simulink model "six_plus_six_AcmsteeringV09_main"  (R2014a)
settings: Solver=FixedStepDiscrete  StartTime=0.0  StopTime=10.0  FixedStep=0.0005  RelTol=1e-3
InitFcn:
  | Veh_Par_wxt
values from neighbouring files (symbols this model uses):
  acc_spdctl = [0 100]    [Veh_Par_wxt.m]
  ag_thr = ecucoder_cal(ag_thr)    [Veh_Par_wxt.m]
  B = 1.8    [Veh_Par_wxt.m]
  bra_em = 100    [Veh_Par_wxt.m]
  bra_pre_gz2 = 100/3    (= 33.3333333333)    [Veh_Par_wxt.m]
  bra_pre_gz34 = 10/3    (= 3.33333333333)    [Veh_Par_wxt.m]
  bra_pre_yd = 10/2    (= 5)    [Veh_Par_wxt.m]
  brakepre_dem_data = [0 1 2 3 4 5 6 7 8 9 10]    [Veh_Par_wxt.m]
  brakeTrq_dem_data = [0 125 251 376 502 627 753 878 1004 1129 1255]    [Veh_Par_wxt.m]
  bratrq_max = 4*1255    (= 5020)    [Veh_Par_wxt.m]
  eff_tran = 0.9    [Veh_Par_wxt.m]
  ESP_switch = ecucoder_cal(ESP_switch)    [Veh_Par_wxt.m]
  G = Mass*g    (= 15696)    [Veh_Par_wxt.m]
  kd1 = ecucoder_cal(kd1)    [Veh_Par_wxt.m]
  kd2 = 0    [Veh_Par_wxt.m]
  ki1 = ecucoder_cal(ki1)    [Veh_Par_wxt.m]
  ki2 = 1    [Veh_Par_wxt.m]
  kp1 = ecucoder_cal(kp1)    [Veh_Par_wxt.m]
  kp2 = 300    [Veh_Par_wxt.m]
  L = L1+L2    (= 2.9)    [Veh_Par_wxt.m]
  premax = 100    [Veh_Par_wxt.m]
  Radius = 0.4572/2    (= 0.2286)    [Veh_Par_wxt.m]
  RC_switch = ecucoder_cal(RC_switch)    [Veh_Par_wxt.m]
  s_opt_yi = 0.15    [Veh_Par_wxt.m]
  s_opt_zhuan = 0.8    [Veh_Par_wxt.m]
  s_opt_zhuan_add = 0.05    [Veh_Par_wxt.m]
  s_opt_zhuan_table = [0.8 0.8 0.3 0.3]    [Veh_Par_wxt.m]
  spd_map_mot = [0 499.85 999.79 1500 2000 2500 3000 3500 4000 4500 4999.8 5999.8]    [Veh_Par_wxt.m]
  spd_spdctl = [0 500]    [Veh_Par_wxt.m]
  speed_thr_park = 5/3.6/Radius*tras_ratio*30/pi    (= 464.143899364)    [Veh_Par_wxt.m]
  TCS_switch = ecucoder_cal(TCS_switch)    [Veh_Par_wxt.m]
  tras_ratio = 8    [Veh_Par_wxt.m]
  trq_map_mot = [70.5 70.012 71.154 65.797 53.917 45.159 38.073 32.685 27.48 17.133 14.949 10.07]    [Veh_Par_wxt.m]
  trqmax_yd = 70.5    [Veh_Par_wxt.m]
  trqmax_zx = 70.5    [Veh_Par_wxt.m]
  trqmaxneg = -70.5    [Veh_Par_wxt.m]
  v_gain = 0.9    [Veh_Par_wxt.m]
  v_table = [0 5 20 100]    [Veh_Par_wxt.m]
  v_thr_park = 5    [Veh_Par_wxt.m]
  zhidong_bianmazhi = [-140000 750000]    [Veh_Par_wxt.m]
  zhidong_down = -140000    [Veh_Par_wxt.m]
  zhidong_up = 750000    [Veh_Par_wxt.m]
  zhidong_youmen = [0 100]    [Veh_Par_wxt.m]
  zhuanxiang_bianmazhi = [-400000 0 400000]    [Veh_Par_wxt.m]
  zhuanxiang_down = -400000    [Veh_Par_wxt.m]
  zhuanxiang_up = 400000    [Veh_Par_wxt.m]
  zhuanxiang_youmen = [-100 0 100]    [Veh_Par_wxt.m]
undefined symbols (not defined in the file or in its folder): ecucoder_acal, guzhang_lf, guzhang_lm, guzhang_lr, guzhang_rf, guzhang_rm, guzhang_rr, myFIS
libraries: simulink x979, ec5744lib x59, fuzblock x2
(part 2 of 26)

== matlab function six_plus_six_AcmsteeringV09_main/MainControl/mode_control/backward/backward/Brake/Switch Case Action Subsystem/MATLAB Function5 ==
  data: bratrq_dem_lf input; bratrq_dem_lm input; bratrq_dem_lr input; bratrq_dem_rf input; bratrq_dem_rm input; bratrq_dem_rr input; pwr_chg_bat input; bratrq_mot_lf output; bratrq_mot_lm output; pwr_chg_bat1 input; pwr_chg_bat2 input; trqlimL_dig_lf input; bratrq_mot_lr output; bratrq_mot_rf output; bratrq_mot_rm output; bratrq_mot_rr output; trqlimL_dig_lm input; trqlimL_dig_lr input; trqlimL_dig_rf input; trqlimL_dig_rm input; trqlimL_dig_rr input; speed_act_lf input; speed_act_lm input; speed_act_lr input; speed_act_rf input; speed_act_rm input; speed_act_rr input; trqlim_map_lf input; brapre_out_l output; brapre_out_r output; trqlim_map_lm input; trqlim_map_lr input; trqlim_map_rf input; trqlim_map_rm input; trqlim_map_rr input; tras_ratio input; guzhang_lf input; guzhang_lm input; guzhang_lr input; guzhang_rf input; guzhang_rm input; guzhang_rr input
function [bratrq_mot_lf,bratrq_mot_lm,bratrq_mot_lr,bratrq_mot_rf,bratrq_mot_rm,bratrq_mot_rr,brapre_out_l,brapre_out_r] = fcn(bratrq_dem_lf,bratrq_dem_lm,bratrq_dem_lr,bratrq_dem_rf,bratrq_dem_rm,bratrq_dem_rr,pwr_chg_bat,pwr_chg_bat1,pwr_chg_bat2,trqlimL_dig_lf,trqlimL_dig_lm,trqlimL_dig_lr,trqlimL_dig_rf,trqlimL_dig_rm,trqlimL_dig_rr,speed_act_lf,speed_act_lm,speed_act_lr,speed_act_rf,speed_act_rm,speed_act_rr,trqlim_map_lf,trqlim_map_lm,trqlim_map_lr,trqlim_map_rf,trqlim_map_rm,trqlim_map_rr,tras_ratio,guzhang_lf,guzhang_lm,guzhang_lr,guzhang_rf,guzhang_rm,guzhang_rr)
%#codegen pid模块在外面做，里面进行十六种情况的判断，先看一下效果，不能再修改。前轴单独控制，后轴低选控制

bratrq_mot_lf1=single(bratrq_dem_lf/tras_ratio);
bratrq_mot_lf2=single(9549*(pwr_chg_bat/2)/speed_act_lf);
bratrq_mot_lf=single(min(trqlimL_dig_lf,min(bratrq_mot_lf1,bratrq_mot_lf2)));

bratrq_mot_lm1=single(bratrq_dem_lm/tras_ratio);
bratrq_mot_lm2=single(9549*(pwr_chg_bat1/2)/speed_act_lm);
bratrq_mot_lm=single(min(trqlimL_dig_lm,min(bratrq_mot_lm1,bratrq_mot_lm2)));

bratrq_mot_lr1=single(bratrq_dem_lr/tras_ratio);
bratrq_mot_lr2=single(9549*(pwr_chg_bat2/2)/speed_act_lr);
bratrq_mot_lr=single(min(trqlimL_dig_lr,min(bratrq_mot_lr1,bratrq_mot_lr2)));
 
bratrq_mot_rf1=single(bratrq_dem_rf/tras_ratio);
bratrq_mot_rf2=single(9549*(pwr_chg_bat/2)/speed_act_rf);
bratrq_mot_rf=single(min(trqlimL_dig_rf,min(bratrq_mot_rf1,bratrq_mot_rf2)));

bratrq_mot_rm1=single(bratrq_dem_rm/tras_ratio);
bratrq_mot_rm2=single(9549*(pwr_chg_bat1/2)/speed_act_rm);
bratrq_mot_rm=single(min(trqlimL_dig_rm,min(bratrq_mot_rm1,bratrq_mot_rm2)));

bratrq_mot_rr1=single(bratrq_dem_rr/tras_ratio);
bratrq_mot_rr2=single(9549*(pwr_chg_bat2/2)/speed_act_rr);
bratrq_mot_rr=single(min(trqlimL_dig_rr,min(bratrq_mot_rr1,bratrq_mot_rr2)));

brapre_out_l=single(((bratrq_dem_lf+bratrq_dem_lm+bratrq_dem_lr)-(bratrq_mot_lf+bratrq_mot_lm+bratrq_mot_lr)*tras_ratio)/3/150);
brapre_out_r=single(((bratrq_dem_rf+bratrq_dem_rm+bratrq_dem_rr)-(bratrq_mot_rf+bratrq_mot_rm+bratrq_mot_rr)*tras_ratio)/3/150);







bratrq_mot_lf=single(min(bratrq_mot_lf,trqlim_map_lf));%限一下最大值在外特性内，最小值大于0
bratrq_mot_lf=single(max(bratrq_mot_lf,0));
bratrq_mot_lr=single(min(bratrq_mot_lr,trqlim_map_lr));
bratrq_mot_lr=single(max(bratrq_mot_lr,0));
bratrq_mot_rf=single(min(bratrq_mot_rf,trqlim_map_rf));
bratrq_mot_rf=single(max(bratrq_mot_rf,0));
bratrq_mot_rr=single(min(bratrq_mot_rr,trqlim_map_rr));
bratrq_mot_rr=single(max(bratrq_mot_rr,0));

% brapre_out_l=brapre_out_l;
% brapre_out_r=brapre_out_r;
brapre_out_l=single(brapre_out_l*150/125);%第二辆车的制动压力与制动力的关系调整一下。
brapre_out_r=single(brapre_out_r*150/125);

if guzhang_lf==1
    bratrq_mot_lf=single(0);
end
if guzhang_lm==1
    bratrq_mot_lm=single(0);
end
if guzhang_lr==1
    bratrq_mot_lr=single(0);
end
if guzhang_rf==1
    bratrq_mot_rf=single(0);
end
if guzhang_rm==1
    bratrq_mot_rm=single(0);
end
if guzhang_rr==1
    bratrq_mot_rr=single(0);
end

end

== system six_plus_six_AcmsteeringV09_main/InputSignalProcess ==
  note: IMU坐标系转换到车辆坐标系
  note: 上坡辅助系统(Hill-start Assist Control，HAC)
  Signals : Inport
  function : TriggerPort  TriggerType=function-call
  Bus Creator : BusCreator  Inputs=8
  Bus Creator1 : BusCreator  Inputs=5
  Bus Creator2 : BusCreator  Inputs=17
  Bus Selector : BusSelector  OutputSignals=RemoteControl,MOTOR,CCM,motec,IMU
  Bus Selector1 : BusSelector  OutputSignals=RemoteControl1,RemoteControl2,RemoteControl3
  Bus Selector2 : BusSelector  OutputSignals=SE,LifeSpan,SH
  Bus Selector3 : BusSelector  OutputSignals=LeftJoystick_UpDown,LeftJoystick_LeftRight,RirhtJoystick_UpDown
  Bus Selector4 : BusSelector  OutputSignals=SA,SD
  Bus Selector6 : BusSelector  OutputSignals=IMU1.Xangularrate,IMU1.Yangularrate,IMU2.Zangularrate,IMU2.Xacceleration,IMU3.Yacceleration,IMU3.Zacceleration,IMU4.NorthSpd,IMU4.SkySpd,IMU5.EastSpd,IMU5.Altitude,IMU6.Longitude,IMU6.Latitude,IMU7.Rolling,IMU7.Heading,IMU8.Pitching
  Compare To Constant : simulink/Logic and Bit Operations/Compare To Constant  relop===  const=7  OutDataTypeStr=boolean
  Compare To Constant1 : simulink/Logic and Bit Operations/Compare To Constant  relop===  const=5  OutDataTypeStr=boolean
  Compare To Constant2 : simulink/Logic and Bit Operations/Compare To Constant  relop===  const=8  OutDataTypeStr=boolean
  Compare To Constant3 : simulink/Logic and Bit Operations/Compare To Constant  relop===  const=8  OutDataTypeStr=boolean
  Compare To Constant4 : simulink/Logic and Bit Operations/Compare To Constant  relop===  const=0  OutDataTypeStr=boolean
  Compare To Constant5 : simulink/Logic and Bit Operations/Compare To Constant  relop===  const=8  OutDataTypeStr=boolean
  Constant : Constant  Value=3  OutDataTypeStr=single  SampleTime=-1
  Constant1 : Constant  Value=0  OutDataTypeStr=single  SampleTime=-1
  Data Type Conversion{,1..16} (17 alike) : DataTypeConversion
  Dead Zone : DeadZone  LowerValue=-1  UpperValue=1  SaturateOnIntegerOverflow=on
  Dead Zone1 : DeadZone  LowerValue=-1  UpperValue=1  SaturateOnIntegerOverflow=on
  Dead Zone2 : DeadZone  LowerValue=0  UpperValue=3  SaturateOnIntegerOverflow=on
  Logical Operator : Logic  Operator=OR  Inputs=3  AllPortsSameDT=off  OutDataTypeStr=boolean
  MATLAB Function : MATLAB Function  TreatAsAtomicUnit=on
  MATLAB Function1 : MATLAB Function  TreatAsAtomicUnit=on
  Memory{,1..3} (4 alike) : Memory  InheritSampleTime=on
  Relational Operator : RelationalOperator  Operator===  OutDataTypeStr=boolean
  Terminator : Terminator
  Terminator1 : Terminator
  Signals_out : Outport
  wires:
  Signals/1 -> Bus Selector/1
  Bus Selector/1 -> Bus Selector1/1  "<RemoteControl>"
  Bus Selector1/1 -> Bus Selector2/1  "<RemoteControl1>"
  Bus Selector2/1 -> Compare To Constant1/1, Compare To Constant4/1, Compare To Constant/1  "<SE>"
  Bus Selector2/2 -> Relational Operator/1, Memory/1  "<LifeSpan>"
  Memory/1 -> Memory1/1
  Compare To Constant/1 -> Logical Operator/1
  Bus Selector1/2 -> Bus Selector3/1  "<RemoteControl2>"
  MATLAB Function/1(acc_dem) -> Dead Zone/1
  MATLAB Function/2(steer_dem) -> Dead Zone1/1
  MATLAB Function/3(brake_dem) -> Dead Zone2/1
  Logical Operator/1 -> Bus Creator/1  "brake_emerg"
  Compare To Constant1/1 -> Bus Creator/2  "park"
  Dead Zone/1 -> Bus Creator/3  "acc_dem"
  Dead Zone1/1 -> Bus Creator/4  "steer_dem"
  Dead Zone2/1 -> Bus Creator/5  "brake_dem"
  Bus Creator/1 -> Bus Creator1/1  "RemoteControl_dem"
  Bus Selector/2 -> Bus Creator1/2  "<MOTOR>"
  Bus Selector/3 -> Bus Creator1/3  "<CCM>"
  Bus Selector1/3 -> Bus Selector4/1  "<RemoteControl3>"
  Bus Selector4/1 -> Compare To Constant2/1  "<SA>"
  Compare To Constant2/1 -> Bus Creator/6  "center"
  Compare To Constant3/1 -> Bus Creator/7  "HAC"
  Bus Creator1/1 -> Signals_out/1
  Bus Selector/4 -> Bus Creator1/4  "<motec>"
  Memory1/1 -> Memory2/1
  Memory2/1 -> Memory3/1
  Memory3/1 -> Relational Operator/2
  Compare To Constant4/1 -> Logical Operator/2
  Compare To Constant5/1 -> Bus Creator/8  "SpdCtl_switch"
  Constant/1 -> Compare To Constant3/1
  Bus Selector2/3 -> Terminator/1  "<SH>"
  Bus Selector4/2 -> Compare To Constant5/1  "<SD>"
  Bus Selector3/3 -> MATLAB Function/3(RirhtJoystick_UpDown)  "<RirhtJoystick_UpDown>"
  Bus Selector3/1 -> MATLAB Function/1(LeftJoystick_UpDown)  "<LeftJoystick_UpDown>"
  Bus Selector3/2 -> MATLAB Function/2(LeftJoystick_LeftRight)  "<LeftJoystick_LeftRight>"
  Constant1/1 -> Logical Operator/3
  Relational Operator/1 -> Terminator1/1
  Bus Creator2/1 -> Bus Creator1/5  "IMU"
  Bus Selector/5 -> Bus Selector6/1  "<IMU>"
  Bus Selector6/1 -> MATLAB Function1/1(Xangularrate)  "<Xangularrate>"
  Bus Selector6/2 -> MATLAB Function1/2(Yangularrate)  "<Yangularrate>"
  Bus Selector6/5 -> MATLAB Function1/5(Yacceleration)  "<Yacceleration>"
  Bus Selector6/6 -> MATLAB Function1/6(Zacceleration)  "<Zacceleration>"
  Bus Selector6/10 -> MATLAB Function1/10(Altitude)  "<Altitude>"
  Bus Selector6/13 -> MATLAB Function1/13(Rolling)  "<Rolling>"
  Bus Selector6/15 -> MATLAB Function1/15(Pitching)  "<Pitching>"
  Bus Selector6/9 -> MATLAB Function1/9(EastSpd)  "<EastSpd>"
  Bus Selector6/12 -> MATLAB Function1/12(Latitude)  "<Latitude>"
  Bus Selector6/8 -> MATLAB Function1/8(SkySpd)  "<SkySpd>"
  Bus Selector6/14 -> MATLAB Function1/14(Heading)  "<Heading>"
  Bus Selector6/11 -> MATLAB Function1/11(Longitude)  "<Longitude>"
  Bus Selector6/4 -> MATLAB Function1/4(Xacceleration)  "<Xacceleration>"
  Bus Selector6/7 -> MATLAB Function1/7(NorthSpd)  "<NorthSpd>"
  Bus Selector6/3 -> MATLAB Function1/3(Zangularrate)  "<Zangularrate>"
  MATLAB Function1/6(Zacceleration1) -> Data Type Conversion5/1
  MATLAB Function1/2(Yangularrate1) -> Data Type Conversion1/1
  MATLAB Function1/7(NorthSpd1) -> Data Type Conversion6/1
  MATLAB Function1/4(Xacceleration1) -> Data Type Conversion3/1
  MATLAB Function1/5(Yacceleration1) -> Data Type Conversion4/1
  MATLAB Function1/10(Altitude1) -> Data Type Conversion9/1
  MATLAB Function1/8(SkySpd1) -> Data Type Conversion7/1
  MATLAB Function1/11(Longitude1) -> Data Type Conversion10/1
  MATLAB Function1/1(Xangularrate1) -> Data Type Conversion/1
  MATLAB Function1/3(Zangularrate1) -> Data Type Conversion2/1
  MATLAB Function1/13(Rolling1) -> Data Type Conversion12/1
  MATLAB Function1/12(Latitude1) -> Data Type Conversion11/1
  MATLAB Function1/9(EastSpd1) -> Data Type Conversion8/1
  MATLAB Function1/15(Pitching1) -> Data Type Conversion14/1
  MATLAB Function1/14(Heading1) -> Data Type Conversion13/1
  MATLAB Function1/17(Yspd) -> Data Type Conversion16/1  "Yspd"
  MATLAB Function1/16(Xspd) -> Data Type Conversion15/1  "Xspd"
  Data Type Conversion/1 -> Bus Creator2/1  "Xangularrate"
  Data Type Conversion1/1 -> Bus Creator2/2  "Yangularrate"
  Data Type Conversion2/1 -> Bus Creator2/3  "Zangularrate"
  Data Type Conversion3/1 -> Bus Creator2/4  "Xacceleration"
  Data Type Conversion4/1 -> Bus Creator2/5  "Yacceleration"
  Data Type Conversion5/1 -> Bus Creator2/6  "Zacceleration"
  Data Type Conversion6/1 -> Bus Creator2/7  "NorthSpd"
  Data Type Conversion7/1 -> Bus Creator2/8  "SkySpd"
  Data Type Conversion8/1 -> Bus Creator2/9  "EastSpd"
  Data Type Conversion9/1 -> Bus Creator2/10  "Altitude"
  Data Type Conversion10/1 -> Bus Creator2/11  "Longitude"
  Data Type Conversion11/1 -> Bus Creator2/12  "Latitude"
  Data Type Conversion12/1 -> Bus Creator2/13  "Rolling"
  Data Type Conversion13/1 -> Bus Creator2/14  "Heading"
  Data Type Conversion14/1 -> Bus Creator2/15  "Pitching"
  Data Type Conversion15/1 -> Bus Creator2/16  "Xspd"
  Data Type Conversion16/1 -> Bus Creator2/17  "Yspd"

== system six_plus_six_AcmsteeringV09_main/MainControl ==
  Signals : Inport
  function : TriggerPort  TriggerType=function-call
  mode_control : Subsystem
  mode_switch : Subsystem
  com_dem : Outport
  wires:
  Signals/1 -> mode_control/2(Signals), mode_switch/1(Signals)
  mode_switch/1(mode_dem_out) -> mode_control/1(mode_dem_out)
  mode_control/1(com_dem) -> com_dem/1

== system six_plus_six_AcmsteeringV09_main/Subsystem ==
  note: ID：电机1为201，电机2为202……
  note: ID：电机1为201，电机2为202……
  note: ID：电机1为201，电机2为202……
  note: ID：电机1为201，电机2为202……
  com_dem : Inport
  Trigger : TriggerPort  TriggerType=function-call  PortDimensions=1
  CANTransmit1 : ec5744lib/RapidECU_U3/04CANCommunication/CANTransmit  canmodule=0  canbuffer=10  canmessageid=hex2dec('C40F327')  canmessagetype=Extended(29-bit ID)  datalength=8  sampletime=-1
  CANTransmit11 : ec5744lib/RapidECU_U3/04CANCommunication/CANTransmit  canmodule=0  canbuffer=12  canmessageid=hex2dec('C40F027')  canmessagetype=Extended(29-bit ID)  datalength=8  sampletime=-1
  CANTransmit12 : ec5744lib/RapidECU_U3/04CANCommunication/CANTransmit  canmodule=0  canbuffer=11  canmessageid=hex2dec('C40F227')  canmessagetype=Extended(29-bit ID)  datalength=8  sampletime=-1
  CANTransmit2 : ec5744lib/RapidECU_U3/04CANCommunication/CANTransmit  canmodule=0  canbuffer=8  canmessageid=hex2dec('C40EF27')  canmessagetype=Extended(29-bit ID)  datalength=8  sampletime=-1
  CANTransmit4 : ec5744lib/RapidECU_U3/04CANCommunication/CANTransmit  canmodule=0  canbuffer=9  canmessageid=hex2dec('C40F127')  canmessagetype=Extended(29-bit ID)  datalength=8  sampletime=-1
  CANTransmit5 : ec5744lib/RapidECU_U3/04CANCommunication/CANTransmit  canmodule=0  canbuffer=13  canmessageid=hex2dec('C40F427')  canmessagetype=Extended(29-bit ID)  datalength=8  sampletime=-1
  CANTransmit6 : ec5744lib/RapidECU_U3/04CANCommunication/CANTransmit  canmodule=1  canbuffer=15  canmessageid=hex2dec('0202')  canmessagetype=Standard(11-bit ID)  datalength=6  sampletime=-1
  CANTransmit7 : ec5744lib/RapidECU_U3/04CANCommunication/CANTransmit  canmodule=1  canbuffer=56  canmessageid=hex2dec('0203')  canmessagetype=Standard(11-bit ID)  datalength=6  sampletime=-1
  CANTransmit8 : ec5744lib/RapidECU_U3/04CANCommunication/CANTransmit  canmodule=1  canbuffer=57  canmessageid=hex2dec('0204')  canmessagetype=Standard(11-bit ID)  datalength=6  sampletime=-1
  CANTransmit9 : ec5744lib/RapidECU_U3/04CANCommunication/CANTransmit  canmodule=1  canbuffer=58  canmessageid=hex2dec('0201')  canmessagetype=Standard(11-bit ID)  datalength=6  sampletime=-1
  Constant{2..3,6,8} (4 alike) : Constant  SampleTime=-1
  Constant{4..5,7,9} (4 alike) : Constant  Value=5  SampleTime=-1
  Data Type Conversion{,1..27} (28 alike) : DataTypeConversion
  Demux : Demux  Outputs=10
  Demux{1..6} (6 alike) : Demux  Outputs=6
  MATLAB Function : MATLAB Function  TreatAsAtomicUnit=on
  MATLAB Function1 : MATLAB Function  TreatAsAtomicUnit=on
  MATLAB Function2 : MATLAB Function  TreatAsAtomicUnit=on
  MATLAB Function3 : MATLAB Function  TreatAsAtomicUnit=on
  Memory{1..3,5} (4 alike) : Memory  InheritSampleTime=on  LinearizeAsDelay=on
  Mux{1..4} (4 alike) : Mux  Inputs=6
  Sum{1..8} (8 alike) : Sum  Inputs=|++
  Terminator{,1..8,10} (10 alike) : Terminator
  VCU1 : Subsystem
  VCU2 : Subsystem
  VCU3 : Subsystem
  VCU4 : Subsystem
  VCU5 : Subsystem
  VCU6 : Subsystem
  wires:
  VCU1/1(output) -> CANTransmit2/1
  CANTransmit2/1 -> Terminator/1
  VCU2/1(output) -> CANTransmit11/1
  CANTransmit11/1 -> Terminator1/1
  VCU3/1(output) -> CANTransmit4/1
  CANTransmit4/1 -> Terminator2/1
  VCU4/1(output) -> CANTransmit12/1
  CANTransmit12/1 -> Terminator3/1
  VCU5/1(output) -> CANTransmit1/1
  CANTransmit1/1 -> Terminator4/1
  VCU6/1(output) -> CANTransmit5/1
  CANTransmit5/1 -> Terminator5/1
  com_dem/1 -> Demux/1
  Demux/1 -> Demux1/1
  Demux1/2 -> VCU1/2(VCU1_CtrlModel_in)
  Demux1/1 -> VCU1/1(VCU1_EnableReq_in)
  Demux1/3 -> VCU1/3(VCU1_GearCmd_in)
  Demux1/4 -> VCU1/4(VCU1_SpeedMax_in)
  Demux1/5 -> VCU1/5(VCU1_TorqueRef_in)
  Demux1/6 -> VCU1/6(VCU1_LifeCnt_in)
  Demux/2 -> Demux2/1
  Demux2/1 -> VCU3/1(VCU1_EnableReq_in)
  Demux2/2 -> VCU3/2(VCU1_CtrlModel_in)
  Demux2/3 -> VCU3/3(VCU1_GearCmd_in)
  Demux2/5 -> VCU3/5(VCU1_TorqueRef_in)
  Demux2/6 -> VCU3/6(VCU1_LifeCnt_in)
  Demux2/4 -> VCU3/4(VCU1_SpeedMax_in)
  Demux3/5 -> VCU5/5(VCU1_TorqueRef_in)
  Demux3/6 -> VCU5/6(VCU1_LifeCnt_in)
  Demux3/4 -> VCU5/4(VCU1_SpeedMax_in)
  Demux3/2 -> VCU5/2(VCU1_CtrlModel_in)
  Demux3/1 -> VCU5/1(VCU1_EnableReq_in)
  Demux3/3 -> VCU5/3(VCU1_GearCmd_in)
  Demux/3 -> Demux3/1
  Demux4/1 -> VCU2/1(VCU1_EnableReq_in)
  Demux4/2 -> VCU2/2(VCU1_CtrlModel_in)
  Demux4/3 -> VCU2/3(VCU1_GearCmd_in)
  Demux4/4 -> VCU2/4(VCU1_SpeedMax_in)
  Demux4/5 -> VCU2/5(VCU1_TorqueRef_in)
  Demux4/6 -> VCU2/6(VCU1_LifeCnt_in)
  Demux/4 -> Demux4/1
  Demux5/3 -> VCU4/3(VCU1_GearCmd_in)
  Demux5/6 -> VCU4/6(VCU1_LifeCnt_in)
  Demux5/5 -> VCU4/5(VCU1_TorqueRef_in)
  Demux5/2 -> VCU4/2(VCU1_CtrlModel_in)
  Demux5/1 -> VCU4/1(VCU1_EnableReq_in)
  Demux5/4 -> VCU4/4(VCU1_SpeedMax_in)
  Demux6/4 -> VCU6/4(VCU1_SpeedMax_in)
  Demux6/1 -> VCU6/1(VCU1_EnableReq_in)
  Demux6/3 -> VCU6/3(VCU1_GearCmd_in)
  Demux6/6 -> VCU6/6(VCU1_LifeCnt_in)
  Demux6/2 -> VCU6/2(VCU1_CtrlModel_in)
  Demux6/5 -> VCU6/5(VCU1_TorqueRef_in)
  Demux/5 -> Demux5/1
  Demux/6 -> Demux6/1
  MATLAB Function/5(position_2) -> Data Type Conversion12/1
  Data Type Conversion2/1 -> Mux1/1
  Constant4/1 -> Sum1/1
  Memory5/1 -> Sum3/2
  Data Type Conversion6/1 -> Mux1/2
  CANTransmit6/1 -> Terminator10/1
  Constant2/1 -> Sum3/1
  MATLAB Function/6(position_1) -> Data Type Conversion9/1
  MATLAB Function/2(zero) -> Data Type Conversion6/1
  Mux1/1 -> CANTransmit6/1
  Sum1/1 -> MATLAB Function/1(data_1)
  MATLAB Function/1(data) -> Data Type Conversion2/1
  MATLAB Function/4(position_3) -> Data Type Conversion14/1
  MATLAB Function/3(position_4) -> Data Type Conversion10/1
  Sum3/1 -> Sum1/2, Memory5/1
  Data Type Conversion10/1 -> Mux1/3
  Data Type Conversion9/1 -> Mux1/6
  Data Type Conversion14/1 -> Mux1/4
  Data Type Conversion12/1 -> Mux1/5
  MATLAB Function1/5(position_2) -> Data Type Conversion3/1
  Data Type Conversion5/1 -> Mux2/1
  Constant5/1 -> Sum2/1
  Memory1/1 -> Sum4/2
  Data Type Conversion7/1 -> Mux2/2
  CANTransmit7/1 -> Terminator6/1
  Constant3/1 -> Sum4/1
  MATLAB Function1/6(position_1) -> Data Type Conversion8/1
  MATLAB Function1/2(zero) -> Data Type Conversion7/1
  Mux2/1 -> CANTransmit7/1
  Sum2/1 -> MATLAB Function1/1(data_1)
  MATLAB Function1/1(data) -> Data Type Conversion5/1
  MATLAB Function1/4(position_3) -> Data Type Conversion4/1
  MATLAB Function1/3(position_4) -> Data Type Conversion1/1
  Sum4/1 -> Memory1/1, Sum2/2
  Data Type Conversion1/1 -> Mux2/3
  Data Type Conversion8/1 -> Mux2/6
  Data Type Conversion4/1 -> Mux2/4
  Data Type Conversion3/1 -> Mux2/5
  MATLAB Function2/5(position_2) -> Data Type Conversion13/1
  Data Type Conversion16/1 -> Mux3/1
  Constant7/1 -> Sum5/1
  Memory2/1 -> Sum6/2
  Data Type Conversion17/1 -> Mux3/2
  CANTransmit8/1 -> Terminator7/1
  Constant6/1 -> Sum6/1
  MATLAB Function2/6(position_1) -> Data Type Conversion18/1
  MATLAB Function2/2(zero) -> Data Type Conversion17/1
  Mux3/1 -> CANTransmit8/1
  Sum5/1 -> MATLAB Function2/1(data_1)
  MATLAB Function2/1(data) -> Data Type Conversion16/1
  MATLAB Function2/4(position_3) -> Data Type Conversion15/1
  MATLAB Function2/3(position_4) -> Data Type Conversion11/1
  Sum6/1 -> Memory2/1, Sum5/2
  Data Type Conversion11/1 -> Mux3/3
  Data Type Conversion18/1 -> Mux3/6
  Data Type Conversion15/1 -> Mux3/4
  Data Type Conversion13/1 -> Mux3/5
  MATLAB Function3/5(position_2) -> Data Type Conversion20/1
  Data Type Conversion22/1 -> Mux4/1
  Constant9/1 -> Sum7/1
  Memory3/1 -> Sum8/2
  Data Type Conversion23/1 -> Mux4/2
  CANTransmit9/1 -> Terminator8/1
  Constant8/1 -> Sum8/1
  MATLAB Function3/6(position_1) -> Data Type Conversion24/1
  MATLAB Function3/2(zero) -> Data Type Conversion23/1
  Mux4/1 -> CANTransmit9/1
  Sum7/1 -> MATLAB Function3/1(data_1)
  MATLAB Function3/1(data) -> Data Type Conversion22/1
  MATLAB Function3/4(position_3) -> Data Type Conversion21/1
  MATLAB Function3/3(position_4) -> Data Type Conversion19/1
  Sum8/1 -> Memory3/1, Sum7/2
  Data Type Conversion19/1 -> Mux4/3
  Data Type Conversion24/1 -> Mux4/6
  Data Type Conversion21/1 -> Mux4/4
  Data Type Conversion20/1 -> Mux4/5
  Demux/9 -> Data Type Conversion26/1  "p3"
  Demux/7 -> Data Type Conversion/1
  Demux/10 -> Data Type Conversion27/1
  Data Type Conversion/1 -> MATLAB Function/2(data_2)
  Data Type Conversion25/1 -> MATLAB Function1/2(data_2)
  Data Type Conversion26/1 -> MATLAB Function2/2(data_2)
  Data Type Conversion27/1 -> MATLAB Function3/2(data_2)
  Demux/8 -> Data Type Conversion25/1

== system six_plus_six_AcmsteeringV09_main/Data_input/1 ==
  In1 : Inport
  In2 : Inport  Port=2
  function : TriggerPort  TriggerType=function-call
  Enabled Subsystem : Subsystem  TreatAsAtomicUnit=on
  motec_spd_2 : Outport
  motec_current_2 : Outport  Port=2
  enable_count : Outport  Port=3
  wires:
  In2/1 -> Enabled Subsystem/1(In2)
  In1/1 -> Enabled Subsystem/Enable
  Enabled Subsystem/1(motec_spd_2) -> motec_spd_2/1
  Enabled Subsystem/2(motec_current_2) -> motec_current_2/1
  Enabled Subsystem/3(enable_count2) -> enable_count/1

== system six_plus_six_AcmsteeringV09_main/Data_input/10 ==
  In1 : Inport
  In2 : Inport  Port=2
  function : TriggerPort  TriggerType=function-call
  Data Type Conversion : DataTypeConversion
  Data Type Conversion1 : DataTypeConversion
  Enabled Subsystem : Subsystem  TreatAsAtomicUnit=on
  Rolling_Out : Outport
  Heading_Out : Outport  Port=2
  wires:
  In1/1 -> Enabled Subsystem/Enable
  In2/1 -> Enabled Subsystem/1(In2)
  Enabled Subsystem/1(Rolling_Out) -> Data Type Conversion/1
  Enabled Subsystem/2(Heading_Out) -> Data Type Conversion1/1
  Data Type Conversion/1 -> Rolling_Out/1
  Data Type Conversion1/1 -> Heading_Out/1

== system six_plus_six_AcmsteeringV09_main/Data_input/11 ==
  In1 : Inport
  In2 : Inport  Port=2
  function : TriggerPort  TriggerType=function-call
  Data Type Conversion : DataTypeConversion
  Enabled Subsystem : Subsystem  TreatAsAtomicUnit=on
  Pitching_Out : Outport
  wires:
  In2/1 -> Enabled Subsystem/1(In2)
  In1/1 -> Enabled Subsystem/Enable
  Enabled Subsystem/1(Pitching_Out) -> Data Type Conversion/1
  Data Type Conversion/1 -> Pitching_Out/1

== system six_plus_six_AcmsteeringV09_main/Data_input/181 ==
  In1 : Inport
  In2 : Inport  Port=2
  function : TriggerPort  TriggerType=function-call
  Enabled Subsystem : Subsystem  TreatAsAtomicUnit=on
  motec_spd_1 : Outport
  motec_current_1 : Outport  Port=2
  enable_count1 : Outport  Port=3
  wires:
  In2/1 -> Enabled Subsystem/1(In2)
  In1/1 -> Enabled Subsystem/Enable
  Enabled Subsystem/1(motec_spd_1) -> motec_spd_1/1
  Enabled Subsystem/2(motec_current_1) -> motec_current_1/1
  Enabled Subsystem/3(enable_count1) -> enable_count1/1

== system six_plus_six_AcmsteeringV09_main/Data_input/2 ==
  In1 : Inport
  In2 : Inport  Port=2
  function : TriggerPort  TriggerType=function-call
  Enabled Subsystem : Subsystem  TreatAsAtomicUnit=on
  motec_spd_4 : Outport
  motec_current_4 : Outport  Port=2
  enable_count : Outport  Port=3
  wires:
  Enabled Subsystem/2(motec_current_4) -> motec_current_4/1
  Enabled Subsystem/1(motec_spd_4) -> motec_spd_4/1
  In1/1 -> Enabled Subsystem/Enable
  In2/1 -> Enabled Subsystem/1(In2)
  Enabled Subsystem/3(enable_count1) -> enable_count/1

== system six_plus_six_AcmsteeringV09_main/Data_input/3 ==
  In1 : Inport
  In2 : Inport  Port=2
  function : TriggerPort  TriggerType=function-call
  Enabled Subsystem : Subsystem  TreatAsAtomicUnit=on
  motec_spd_3 : Outport
  motec_current_3 : Outport  Port=2
  enable_count3 : Outport  Port=3
  wires:
  Enabled Subsystem/2(motec_current_3) -> motec_current_3/1
  Enabled Subsystem/1(motec_spd_3) -> motec_spd_3/1
  In1/1 -> Enabled Subsystem/Enable
  In2/1 -> Enabled Subsystem/1(In2)
  Enabled Subsystem/3(enable_count1) -> enable_count3/1

== system six_plus_six_AcmsteeringV09_main/Data_input/4 ==
  In1 : Inport
  In2 : Inport  Port=2
  function : TriggerPort  TriggerType=function-call
  Data Type Conversion : DataTypeConversion
  Data Type Conversion1 : DataTypeConversion
  Enabled Subsystem : Subsystem  TreatAsAtomicUnit=on
  Xangularrate_Out : Outport
  Yangularrate_Out : Outport  Port=2
  wires:
  In2/1 -> Enabled Subsystem/1(In2)
  In1/1 -> Enabled Subsystem/Enable
  Enabled Subsystem/1(Xangularrate_Out) -> Data Type Conversion/1
  Enabled Subsystem/2(Yangularrate_Out) -> Data Type Conversion1/1
  Data Type Conversion/1 -> Xangularrate_Out/1
  Data Type Conversion1/1 -> Yangularrate_Out/1

== system six_plus_six_AcmsteeringV09_main/Data_input/5 ==
  In1 : Inport
  In2 : Inport  Port=2
  function : TriggerPort  TriggerType=function-call
  Data Type Conversion : DataTypeConversion
  Data Type Conversion1 : DataTypeConversion
  Enabled Subsystem : Subsystem  TreatAsAtomicUnit=on
  Zangularrate_Out : Outport
  Xacceleration_Out : Outport  Port=2
  wires:
  Enabled Subsystem/2(Xacceleration_Out) -> Data Type Conversion1/1
  Enabled Subsystem/1(Zangularrate_Out) -> Data Type Conversion/1
  In1/1 -> Enabled Subsystem/Enable
  In2/1 -> Enabled Subsystem/1(In2)
  Data Type Conversion/1 -> Zangularrate_Out/1
  Data Type Conversion1/1 -> Xacceleration_Out/1

== system six_plus_six_AcmsteeringV09_main/Data_input/6 ==
  In1 : Inport
  In2 : Inport  Port=2
  function : TriggerPort  TriggerType=function-call
  Data Type Conversion : DataTypeConversion
  Data Type Conversion1 : DataTypeConversion
  Enabled Subsystem : Subsystem  TreatAsAtomicUnit=on
  Yacceleration_Out : Outport
  Zacceleration_Out : Outport  Port=2
  wires:
  In2/1 -> Enabled Subsystem/1(In2)
  In1/1 -> Enabled Subsystem/Enable
  Enabled Subsystem/1(Yacceleration_Out) -> Data Type Conversion/1
  Enabled Subsystem/2(Zacceleration_Out) -> Data Type Conversion1/1
  Data Type Conversion/1 -> Yacceleration_Out/1
  Data Type Conversion1/1 -> Zacceleration_Out/1

== system six_plus_six_AcmsteeringV09_main/Data_input/7 ==
  In1 : Inport
  In2 : Inport  Port=2
  function : TriggerPort  TriggerType=function-call
  Data Type Conversion : DataTypeConversion
  Data Type Conversion1 : DataTypeConversion
  Enabled Subsystem : Subsystem  TreatAsAtomicUnit=on
  NorthSpd_Out : Outport
  SkySpd_Out : Outport  Port=2
  wires:
  In1/1 -> Enabled Subsystem/Enable
  In2/1 -> Enabled Subsystem/1(In2)
  Enabled Subsystem/1(NorthSpd_Out) -> Data Type Conversion/1
  Enabled Subsystem/2(SkySpd_Out) -> Data Type Conversion1/1
  Data Type Conversion1/1 -> SkySpd_Out/1
  Data Type Conversion/1 -> NorthSpd_Out/1

== system six_plus_six_AcmsteeringV09_main/Data_input/8 ==
  In1 : Inport
  In2 : Inport  Port=2
  function : TriggerPort  TriggerType=function-call
  Data Type Conversion : DataTypeConversion
  Data Type Conversion1 : DataTypeConversion
  Enabled Subsystem : Subsystem  TreatAsAtomicUnit=on
  EastSpd_Out : Outport
  Altitude_Out : Outport  Port=2
  wires:
  Enabled Subsystem/2(Altitude_Out) -> Data Type Conversion1/1
  Enabled Subsystem/1(EastSpd_Out) -> Data Type Conversion/1
  In2/1 -> Enabled Subsystem/1(In2)
  In1/1 -> Enabled Subsystem/Enable
  Data Type Conversion1/1 -> Altitude_Out/1
  Data Type Conversion/1 -> EastSpd_Out/1

== system six_plus_six_AcmsteeringV09_main/Data_input/9 ==
  In1 : Inport
  In2 : Inport  Port=2
  function : TriggerPort  TriggerType=function-call
  Data Type Conversion : DataTypeConversion
  Data Type Conversion1 : DataTypeConversion
  Enabled Subsystem : Subsystem  TreatAsAtomicUnit=on
  Longitude_Out : Outport
  Latitude_Out : Outport  Port=2
  wires:
  In1/1 -> Enabled Subsystem/Enable
  In2/1 -> Enabled Subsystem/1(In2)
  Enabled Subsystem/1(Longitude_Out) -> Data Type Conversion/1
  Enabled Subsystem/2(Latitude_Out) -> Data Type Conversion1/1
  Data Type Conversion/1 -> Longitude_Out/1
  Data Type Conversion1/1 -> Latitude_Out/1

== system six_plus_six_AcmsteeringV09_main/Data_input/BMS1 ==
  In1 : Inport
  In2 : Inport  Port=2
  Trigger : TriggerPort  TriggerType=function-call  PortDimensions=1
  BMS1 : Subsystem
  BMS1_TotalVol : Outport
  BMS1_TotalCurrent : Outport  Port=2
  BMS1_Sys_Status2 : Outport  Port=3
  BMS1_Sys_Status1 : Outport  Port=4
  BMS1_SOC : Outport  Port=5
  wires:
  In2/1 -> BMS1/1(input)
  In1/1 -> BMS1/Enable
  BMS1/1(BMS1_TotalVol_Out) -> BMS1_TotalVol/1
  BMS1/4(BMS1_Sys_Status1_Out) -> BMS1_Sys_Status1/1
  BMS1/3(BMS1_Sys_Status2_Out) -> BMS1_Sys_Status2/1
  BMS1/5(BMS1_SOC_Out) -> BMS1_SOC/1
  BMS1/2(BMS1_TotalCurrent_Out) -> BMS1_TotalCurrent/1

== system six_plus_six_AcmsteeringV09_main/Data_input/BMS1-2 ==
  In1 : Inport
  In2 : Inport  Port=2
  Trigger : TriggerPort  TriggerType=function-call  PortDimensions=1
  BMS1 : Subsystem
  BMS1_TotalVol : Outport
  BMS1_TotalCurrent : Outport  Port=2
  BMS1_Sys_Status2 : Outport  Port=3
  BMS1_Sys_Status1 : Outport  Port=4
  BMS1_SOC : Outport  Port=5
  wires:
  In2/1 -> BMS1/1(input)
  In1/1 -> BMS1/Enable
  BMS1/1(BMS1_TotalVol_Out) -> BMS1_TotalVol/1
  BMS1/4(BMS1_Sys_Status1_Out) -> BMS1_Sys_Status1/1
  BMS1/3(BMS1_Sys_Status2_Out) -> BMS1_Sys_Status2/1
  BMS1/5(BMS1_SOC_Out) -> BMS1_SOC/1
  BMS1/2(BMS1_TotalCurrent_Out) -> BMS1_TotalCurrent/1

== system six_plus_six_AcmsteeringV09_main/Data_input/BMS1_1 ==
  In1 : Inport
  In2 : Inport  Port=2
  Trigger : TriggerPort  TriggerType=function-call  PortDimensions=1
  BMS1 : Subsystem
  BMS1_TotalVol : Outport
  BMS1_TotalCurrent : Outport  Port=2
  BMS1_Sys_Status2 : Outport  Port=3
  BMS1_Sys_Status1 : Outport  Port=4
  BMS1_SOC : Outport  Port=5
  wires:
  In2/1 -> BMS1/1(input)
  In1/1 -> BMS1/Enable
  BMS1/1(BMS1_TotalVol_Out) -> BMS1_TotalVol/1
  BMS1/4(BMS1_Sys_Status1_Out) -> BMS1_Sys_Status1/1
  BMS1/3(BMS1_Sys_Status2_Out) -> BMS1_Sys_Status2/1
  BMS1/5(BMS1_SOC_Out) -> BMS1_SOC/1
  BMS1/2(BMS1_TotalCurrent_Out) -> BMS1_TotalCurrent/1

== system six_plus_six_AcmsteeringV09_main/Data_input/BMS2 ==
  In1 : Inport
  In2 : Inport  Port=2
  Trigger : TriggerPort  TriggerType=function-call  PortDimensions=1
  BMS2 : Subsystem
  BMS2_LowSingleVol : Outport
  BMS2_HighSingleVol : Outport  Port=2
  wires:
  BMS2/2(BMS2_HighSingleVol_Out) -> BMS2_HighSingleVol/1
  BMS2/1(BMS2_LowSingleVol_Out) -> BMS2_LowSingleVol/1
  In1/1 -> BMS2/Enable
  In2/1 -> BMS2/1(input)

== system six_plus_six_AcmsteeringV09_main/Data_input/BMS2_1 ==
  In1 : Inport
  In2 : Inport  Port=2
  Trigger : TriggerPort  TriggerType=function-call  PortDimensions=1
  BMS2 : Subsystem
  BMS2_LowSingleVol : Outport
  BMS2_HighSingleVol : Outport  Port=2
  wires:
  BMS2/2(BMS2_HighSingleVol_Out) -> BMS2_HighSingleVol/1
  BMS2/1(BMS2_LowSingleVol_Out) -> BMS2_LowSingleVol/1
  In1/1 -> BMS2/Enable
  In2/1 -> BMS2/1(input)

== system six_plus_six_AcmsteeringV09_main/Data_input/BMS2_2 ==
  In1 : Inport
  In2 : Inport  Port=2
  Trigger : TriggerPort  TriggerType=function-call  PortDimensions=1
  BMS2 : Subsystem
  BMS2_LowSingleVol : Outport
  BMS2_HighSingleVol : Outport  Port=2
  wires:
  BMS2/2(BMS2_HighSingleVol_Out) -> BMS2_HighSingleVol/1
  BMS2/1(BMS2_LowSingleVol_Out) -> BMS2_LowSingleVol/1
  In1/1 -> BMS2/Enable
  In2/1 -> BMS2/1(input)

== system six_plus_six_AcmsteeringV09_main/Data_input/BMS3 ==
  In1 : Inport
  In2 : Inport  Port=2
  Trigger : TriggerPort  TriggerType=function-call  PortDimensions=1
  BMS3 : Subsystem
  BMS3_LowTemperature : Outport
  BMS3_HighTemperature : Outport  Port=2
  wires:
  In2/1 -> BMS3/1(input)
  BMS3/2(BMS3_HighTemperature_Out) -> BMS3_HighTemperature/1
  BMS3/1(BMS3_LowTemperature_Out) -> BMS3_LowTemperature/1
  In1/1 -> BMS3/Enable

== system six_plus_six_AcmsteeringV09_main/Data_input/BMS3_1 ==
  In1 : Inport
  In2 : Inport  Port=2
  Trigger : TriggerPort  TriggerType=function-call  PortDimensions=1
  BMS3 : Subsystem
  BMS3_LowTemperature : Outport
  BMS3_HighTemperature : Outport  Port=2
  wires:
  In2/1 -> BMS3/1(input)
  BMS3/2(BMS3_HighTemperature_Out) -> BMS3_HighTemperature/1
  BMS3/1(BMS3_LowTemperature_Out) -> BMS3_LowTemperature/1
  In1/1 -> BMS3/Enable

== system six_plus_six_AcmsteeringV09_main/Data_input/BMS3_2 ==
  In1 : Inport
  In2 : Inport  Port=2
  Trigger : TriggerPort  TriggerType=function-call  PortDimensions=1
  BMS3 : Subsystem
  BMS3_LowTemperature : Outport
  BMS3_HighTemperature : Outport  Port=2
  wires:
  In2/1 -> BMS3/1(input)
  BMS3/2(BMS3_HighTemperature_Out) -> BMS3_HighTemperature/1
  BMS3/1(BMS3_LowTemperature_Out) -> BMS3_LowTemperature/1
  In1/1 -> BMS3/Enable

== system six_plus_six_AcmsteeringV09_main/Data_input/BMS4 ==
  In1 : Inport
  In2 : Inport  Port=2
  Trigger : TriggerPort  TriggerType=function-call  PortDimensions=1
  BMS4 : Subsystem
  BMS4_Sys_Status : Outport
  BMS4_InputVolKEYON : Outport  Port=2
  BMS4_InputVolCHG : Outport  Port=3
  BMS4_InputVolACC : Outport  Port=4
  wires:
  In2/1 -> BMS4/1(input)
  BMS4/2(BMS4_InputVolKEYON_Out) -> BMS4_InputVolKEYON/1
  In1/1 -> BMS4/Enable
  BMS4/4(BMS4_InputVolACC_Out) -> BMS4_InputVolACC/1
  BMS4/1(BMS4_Sys_Status3_Out) -> BMS4_Sys_Status/1
  BMS4/3(BMS4_InputVolCHG_Out) -> BMS4_InputVolCHG/1

== system six_plus_six_AcmsteeringV09_main/Data_input/BMS4_1 ==
  In1 : Inport
  In2 : Inport  Port=2
  Trigger : TriggerPort  TriggerType=function-call  PortDimensions=1
  BMS4 : Subsystem
  BMS4_Sys_Status : Outport
  BMS4_InputVolKEYON : Outport  Port=2
  BMS4_InputVolCHG : Outport  Port=3
  BMS4_InputVolACC : Outport  Port=4
  wires:
  In2/1 -> BMS4/1(input)
  BMS4/2(BMS4_InputVolKEYON_Out) -> BMS4_InputVolKEYON/1
  In1/1 -> BMS4/Enable
  BMS4/4(BMS4_InputVolACC_Out) -> BMS4_InputVolACC/1
  BMS4/1(BMS4_Sys_Status3_Out) -> BMS4_Sys_Status/1
  BMS4/3(BMS4_InputVolCHG_Out) -> BMS4_InputVolCHG/1

== system six_plus_six_AcmsteeringV09_main/Data_input/BMS4_2 ==
  In1 : Inport
  In2 : Inport  Port=2
  Trigger : TriggerPort  TriggerType=function-call  PortDimensions=1
  BMS4 : Subsystem
  BMS4_Sys_Status : Outport
  BMS4_InputVolKEYON : Outport  Port=2
  BMS4_InputVolCHG : Outport  Port=3
  BMS4_InputVolACC : Outport  Port=4
  wires:
  In2/1 -> BMS4/1(input)
  BMS4/2(BMS4_InputVolKEYON_Out) -> BMS4_InputVolKEYON/1
  In1/1 -> BMS4/Enable
  BMS4/4(BMS4_InputVolACC_Out) -> BMS4_InputVolACC/1
  BMS4/1(BMS4_Sys_Status3_Out) -> BMS4_Sys_Status/1
  BMS4/3(BMS4_InputVolCHG_Out) -> BMS4_InputVolCHG/1

== system six_plus_six_AcmsteeringV09_main/Data_input/BMS5 ==
  In1 : Inport
  In2 : Inport  Port=2
  Trigger : TriggerPort  TriggerType=function-call  PortDimensions=1
  BMS5 : Subsystem
  BMS5_UpDownReuest : Outport
  BMS5_FeedbackPower : Outport  Port=2
  BMS5_FailureLevel : Outport  Port=3
  BMS5_ContDischargePower : Outport  Port=4
  BMS5_15s_InstanceDisPower : Outport  Port=5
  wires:
  BMS5/5(BMS5_15s_InstanceDisPower_Out) -> BMS5_15s_InstanceDisPower/1
  BMS5/1(BMS5_UpDownRequest_Out) -> BMS5_UpDownReuest/1
  In2/1 -> BMS5/1(input)
  BMS5/4(BMS5_ContDischargePower_Out) -> BMS5_ContDischargePower/1
  BMS5/2(BMS5_FeedbackPower_Out) -> BMS5_FeedbackPower/1
  BMS5/3(BMS5_FailureLevel_Out) -> BMS5_FailureLevel/1
  In1/1 -> BMS5/Enable

== system six_plus_six_AcmsteeringV09_main/Data_input/BMS5_1 ==
  In1 : Inport
  In2 : Inport  Port=2
  Trigger : TriggerPort  TriggerType=function-call  PortDimensions=1
  BMS5 : Subsystem
  BMS5_UpDownReuest : Outport
  BMS5_FeedbackPower : Outport  Port=2
  BMS5_FailureLevel : Outport  Port=3
  BMS5_ContDischargePower : Outport  Port=4
  BMS5_15s_InstanceDisPower : Outport  Port=5
  wires:
  BMS5/5(BMS5_15s_InstanceDisPower_Out) -> BMS5_15s_InstanceDisPower/1
  BMS5/1(BMS5_UpDownRequest_Out) -> BMS5_UpDownReuest/1
  In2/1 -> BMS5/1(input)
  BMS5/4(BMS5_ContDischargePower_Out) -> BMS5_ContDischargePower/1
  BMS5/2(BMS5_FeedbackPower_Out) -> BMS5_FeedbackPower/1
  BMS5/3(BMS5_FailureLevel_Out) -> BMS5_FailureLevel/1
  In1/1 -> BMS5/Enable

== system six_plus_six_AcmsteeringV09_main/Data_input/BMS5_2 ==
  In1 : Inport
  In2 : Inport  Port=2
  Trigger : TriggerPort  TriggerType=function-call  PortDimensions=1
  BMS5 : Subsystem
  BMS5_UpDownReuest : Outport
  BMS5_FeedbackPower : Outport  Port=2
  BMS5_FailureLevel : Outport  Port=3
  BMS5_ContDischargePower : Outport  Port=4
  BMS5_15s_InstanceDisPower : Outport  Port=5
  wires:
  BMS5/5(BMS5_15s_InstanceDisPower_Out) -> BMS5_15s_InstanceDisPower/1
  BMS5/1(BMS5_UpDownRequest_Out) -> BMS5_UpDownReuest/1
  In2/1 -> BMS5/1(input)
  BMS5/4(BMS5_ContDischargePower_Out) -> BMS5_ContDischargePower/1
  BMS5/2(BMS5_FeedbackPower_Out) -> BMS5_FeedbackPower/1
  BMS5/3(BMS5_FailureLevel_Out) -> BMS5_FailureLevel/1
  In1/1 -> BMS5/Enable

== system six_plus_six_AcmsteeringV09_main/Data_input/Enabled Subsystem ==
  In1 : Inport
  Enable : EnablePort
  Subsystem : Subsystem
  Out1 : Outport
  wires:
  In1/1 -> Out1/1

== system six_plus_six_AcmsteeringV09_main/Data_input/MCU0 ==
  In1 : Inport
  In2 : Inport  Port=2
  Trigger : TriggerPort  TriggerType=function-call  PortDimensions=1
  MCU0 : Subsystem
  MCU0_TorqueMax : Outport
  MCU0_EmergShutDown : Outport  Port=2
  MCU_ShutDownAllow : Outport  Port=3
  MCU_HighVol : Outport  Port=4
  MCU0_LiftCnt : Outport  Port=5
  MCU0_torqueFdk : Outport  Port=6
  MCU0_SpeedFdk : Outport  Port=7
  MCU0_GearStatus : Outport  Port=8
  MCU0_ControlMode : Outport  Port=9
  MCU0_WorkStatus : Outport  Port=10
  wires:
  In2/1 -> MCU0/1(input)
  In1/1 -> MCU0/Enable
  MCU0/1(MCU0_TorqueMax_Out) -> MCU0_TorqueMax/1
  MCU0/2(MCU0_EmergShutDown_Out) -> MCU0_EmergShutDown/1
  MCU0/5(MCU0_LiftCnt_Out) -> MCU0_LiftCnt/1
  MCU0/6(MCU0_TorqueFdk_Out) -> MCU0_torqueFdk/1
  MCU0/7(MCU0_SpeedFdk_Out) -> MCU0_SpeedFdk/1
  MCU0/3(MCU0_ShutDowAllow_Out) -> MCU_ShutDownAllow/1
  MCU0/4(MCU0_HighVol_Out) -> MCU_HighVol/1
  MCU0/10(MCU0_WorkStatus_Out) -> MCU0_WorkStatus/1
  MCU0/8(MCU0_GearStatus_Out) -> MCU0_GearStatus/1
  MCU0/9(MCU0_ControlMode_Out) -> MCU0_ControlMode/1

== system six_plus_six_AcmsteeringV09_main/Data_input/MCU0_1 ==
  In1 : Inport
  In2 : Inport  Port=2
  Trigger : TriggerPort  TriggerType=function-call  PortDimensions=1
  MCU0 : Subsystem
  MCU0_TorqueMax : Outport
  MCU0_EmergShutDown : Outport  Port=2
  MCU_ShutDownAllow : Outport  Port=3
  MCU_HighVol : Outport  Port=4
  MCU0_LiftCnt : Outport  Port=5
  MCU0_torqueFdk : Outport  Port=6
  MCU0_SpeedFdk : Outport  Port=7
  MCU0_GearStatus : Outport  Port=8
  MCU0_ControlMode : Outport  Port=9
  MCU0_WorkStatus : Outport  Port=10
  wires:
  In2/1 -> MCU0/1(input)
  In1/1 -> MCU0/Enable
  MCU0/1(MCU0_TorqueMax_Out) -> MCU0_TorqueMax/1
  MCU0/2(MCU0_EmergShutDown_Out) -> MCU0_EmergShutDown/1
  MCU0/5(MCU0_LiftCnt_Out) -> MCU0_LiftCnt/1
  MCU0/6(MCU0_TorqueFdk_Out) -> MCU0_torqueFdk/1
  MCU0/7(MCU0_SpeedFdk_Out) -> MCU0_SpeedFdk/1
  MCU0/3(MCU0_ShutDowAllow_Out) -> MCU_ShutDownAllow/1
  MCU0/4(MCU0_HighVol_Out) -> MCU_HighVol/1
  MCU0/10(MCU0_WorkStatus_Out) -> MCU0_WorkStatus/1
  MCU0/8(MCU0_GearStatus_Out) -> MCU0_GearStatus/1
  MCU0/9(MCU0_ControlMode_Out) -> MCU0_ControlMode/1

== system six_plus_six_AcmsteeringV09_main/Data_input/MCU0_2 ==
  In1 : Inport
  In2 : Inport  Port=2
  Trigger : TriggerPort  TriggerType=function-call  PortDimensions=1
  MCU0 : Subsystem
  MCU0_TorqueMax : Outport
  MCU0_EmergShutDown : Outport  Port=2
  MCU_ShutDownAllow : Outport  Port=3
  MCU_HighVol : Outport  Port=4
  MCU0_LiftCnt : Outport  Port=5
  MCU0_torqueFdk : Outport  Port=6
  MCU0_SpeedFdk : Outport  Port=7
  MCU0_GearStatus : Outport  Port=8
  MCU0_ControlMode : Outport  Port=9
  MCU0_WorkStatus : Outport  Port=10
  wires:
  In2/1 -> MCU0/1(input)
  In1/1 -> MCU0/Enable
  MCU0/1(MCU0_TorqueMax_Out) -> MCU0_TorqueMax/1
  MCU0/2(MCU0_EmergShutDown_Out) -> MCU0_EmergShutDown/1
  MCU0/5(MCU0_LiftCnt_Out) -> MCU0_LiftCnt/1
  MCU0/6(MCU0_TorqueFdk_Out) -> MCU0_torqueFdk/1
  MCU0/7(MCU0_SpeedFdk_Out) -> MCU0_SpeedFdk/1
  MCU0/3(MCU0_ShutDowAllow_Out) -> MCU_ShutDownAllow/1
  MCU0/4(MCU0_HighVol_Out) -> MCU_HighVol/1
  MCU0/10(MCU0_WorkStatus_Out) -> MCU0_WorkStatus/1
  MCU0/8(MCU0_GearStatus_Out) -> MCU0_GearStatus/1
  MCU0/9(MCU0_ControlMode_Out) -> MCU0_ControlMode/1

== system six_plus_six_AcmsteeringV09_main/Data_input/MCU0_3 ==
  In1 : Inport
  In2 : Inport  Port=2
  Trigger : TriggerPort  TriggerType=function-call  PortDimensions=1
  MCU0 : Subsystem
  MCU0_TorqueMax : Outport
  MCU0_EmergShutDown : Outport  Port=2
  MCU_ShutDownAllow : Outport  Port=3
  MCU_HighVol : Outport  Port=4
  MCU0_LiftCnt : Outport  Port=5
  MCU0_torqueFdk : Outport  Port=6
  MCU0_SpeedFdk : Outport  Port=7
  MCU0_GearStatus : Outport  Port=8
  MCU0_ControlMode : Outport  Port=9
  MCU0_WorkStatus : Outport  Port=10
  wires:
  In2/1 -> MCU0/1(input)
  In1/1 -> MCU0/Enable
  MCU0/1(MCU0_TorqueMax_Out) -> MCU0_TorqueMax/1
  MCU0/2(MCU0_EmergShutDown_Out) -> MCU0_EmergShutDown/1
  MCU0/5(MCU0_LiftCnt_Out) -> MCU0_LiftCnt/1
  MCU0/6(MCU0_TorqueFdk_Out) -> MCU0_torqueFdk/1
  MCU0/7(MCU0_SpeedFdk_Out) -> MCU0_SpeedFdk/1
  MCU0/3(MCU0_ShutDowAllow_Out) -> MCU_ShutDownAllow/1
  MCU0/4(MCU0_HighVol_Out) -> MCU_HighVol/1
  MCU0/10(MCU0_WorkStatus_Out) -> MCU0_WorkStatus/1
  MCU0/8(MCU0_GearStatus_Out) -> MCU0_GearStatus/1
  MCU0/9(MCU0_ControlMode_Out) -> MCU0_ControlMode/1

== system six_plus_six_AcmsteeringV09_main/Data_input/MCU0_4 ==
  In1 : Inport
  In2 : Inport  Port=2
  Trigger : TriggerPort  TriggerType=function-call  PortDimensions=1
  MCU0 : Subsystem
  MCU0_TorqueMax : Outport
  MCU0_EmergShutDown : Outport  Port=2
  MCU_ShutDownAllow : Outport  Port=3
  MCU_HighVol : Outport  Port=4
  MCU0_LiftCnt : Outport  Port=5
  MCU0_torqueFdk : Outport  Port=6
  MCU0_SpeedFdk : Outport  Port=7
  MCU0_GearStatus : Outport  Port=8
  MCU0_ControlMode : Outport  Port=9
  MCU0_WorkStatus : Outport  Port=10
  wires:
  In2/1 -> MCU0/1(input)
  In1/1 -> MCU0/Enable
  MCU0/1(MCU0_TorqueMax_Out) -> MCU0_TorqueMax/1
  MCU0/2(MCU0_EmergShutDown_Out) -> MCU0_EmergShutDown/1
  MCU0/5(MCU0_LiftCnt_Out) -> MCU0_LiftCnt/1
  MCU0/6(MCU0_TorqueFdk_Out) -> MCU0_torqueFdk/1
  MCU0/7(MCU0_SpeedFdk_Out) -> MCU0_SpeedFdk/1
  MCU0/3(MCU0_ShutDowAllow_Out) -> MCU_ShutDownAllow/1
  MCU0/4(MCU0_HighVol_Out) -> MCU_HighVol/1
  MCU0/10(MCU0_WorkStatus_Out) -> MCU0_WorkStatus/1
  MCU0/8(MCU0_GearStatus_Out) -> MCU0_GearStatus/1
  MCU0/9(MCU0_ControlMode_Out) -> MCU0_ControlMode/1

== system six_plus_six_AcmsteeringV09_main/Data_input/MCU0_5 ==
  In1 : Inport
  In2 : Inport  Port=2
  Trigger : TriggerPort  TriggerType=function-call  PortDimensions=1
  MCU0 : Subsystem
  MCU0_TorqueMax : Outport
  MCU0_EmergShutDown : Outport  Port=2
  MCU_ShutDownAllow : Outport  Port=3
  MCU_HighVol : Outport  Port=4
  MCU0_LiftCnt : Outport  Port=5
  MCU0_torqueFdk : Outport  Port=6
  MCU0_SpeedFdk : Outport  Port=7
  MCU0_GearStatus : Outport  Port=8
  MCU0_ControlMode : Outport  Port=9
  MCU0_WorkStatus : Outport  Port=10
  wires:
  In2/1 -> MCU0/1(input)
  In1/1 -> MCU0/Enable
  MCU0/1(MCU0_TorqueMax_Out) -> MCU0_TorqueMax/1
  MCU0/2(MCU0_EmergShutDown_Out) -> MCU0_EmergShutDown/1
  MCU0/5(MCU0_LiftCnt_Out) -> MCU0_LiftCnt/1
  MCU0/6(MCU0_TorqueFdk_Out) -> MCU0_torqueFdk/1
  MCU0/7(MCU0_SpeedFdk_Out) -> MCU0_SpeedFdk/1
  MCU0/3(MCU0_ShutDowAllow_Out) -> MCU_ShutDownAllow/1
  MCU0/4(MCU0_HighVol_Out) -> MCU_HighVol/1
  MCU0/10(MCU0_WorkStatus_Out) -> MCU0_WorkStatus/1
  MCU0/8(MCU0_GearStatus_Out) -> MCU0_GearStatus/1
  MCU0/9(MCU0_ControlMode_Out) -> MCU0_ControlMode/1

== system six_plus_six_AcmsteeringV09_main/Data_input/MCU1 ==
  In1 : Inport
  In2 : Inport  Port=2
  Trigger : TriggerPort  TriggerType=function-call  PortDimensions=1
  MCU1 : Subsystem
  MCU1_ControlTemp : Outport
  MCU1_MotorTemp : Outport  Port=2
  MCU_PowerFdk : Outport  Port=3
  MCU1_idc : Outport  Port=4
  MCU_Udc : Outport  Port=5
  wires:
  MCU1/2(MCU1_MotorTemp_Out) -> MCU1_MotorTemp/1
  In1/1 -> MCU1/Enable
  MCU1/1(MCU1_ControlTemp_Out) -> MCU1_ControlTemp/1
  MCU1/4(MCU1_Idc_Out) -> MCU1_idc/1
  MCU1/5(MCU1_Udc_Out) -> MCU_Udc/1
  In2/1 -> MCU1/1(input)
  MCU1/3(MCU1_PowerFdk_Out) -> MCU_PowerFdk/1

== system six_plus_six_AcmsteeringV09_main/Data_input/MCU1_1 ==
  In1 : Inport
  In2 : Inport  Port=2
  Trigger : TriggerPort  TriggerType=function-call  PortDimensions=1
  MCU1 : Subsystem
  MCU1_ControlTemp : Outport
  MCU1_MotorTemp : Outport  Port=2
  MCU_PowerFdk : Outport  Port=3
  MCU1_idc : Outport  Port=4
  MCU_Udc : Outport  Port=5
  wires:
  MCU1/2(MCU1_MotorTemp_Out) -> MCU1_MotorTemp/1
  In1/1 -> MCU1/Enable
  MCU1/1(MCU1_ControlTemp_Out) -> MCU1_ControlTemp/1
  MCU1/4(MCU1_Idc_Out) -> MCU1_idc/1
  MCU1/5(MCU1_Udc_Out) -> MCU_Udc/1
  In2/1 -> MCU1/1(input)
  MCU1/3(MCU1_PowerFdk_Out) -> MCU_PowerFdk/1

== system six_plus_six_AcmsteeringV09_main/Data_input/MCU1_2 ==
  In1 : Inport
  In2 : Inport  Port=2
  Trigger : TriggerPort  TriggerType=function-call  PortDimensions=1
  MCU1 : Subsystem
  MCU1_ControlTemp : Outport
  MCU1_MotorTemp : Outport  Port=2
  MCU_PowerFdk : Outport  Port=3
  MCU1_idc : Outport  Port=4
  MCU_Udc : Outport  Port=5
  wires:
  MCU1/2(MCU1_MotorTemp_Out) -> MCU1_MotorTemp/1
  In1/1 -> MCU1/Enable
  MCU1/1(MCU1_ControlTemp_Out) -> MCU1_ControlTemp/1
  MCU1/4(MCU1_Idc_Out) -> MCU1_idc/1
  MCU1/5(MCU1_Udc_Out) -> MCU_Udc/1
  In2/1 -> MCU1/1(input)
  MCU1/3(MCU1_PowerFdk_Out) -> MCU_PowerFdk/1

== system six_plus_six_AcmsteeringV09_main/Data_input/MCU1_3 ==
  In1 : Inport
  In2 : Inport  Port=2
  Trigger : TriggerPort  TriggerType=function-call  PortDimensions=1
  MCU1 : Subsystem
  MCU1_ControlTemp : Outport
  MCU1_MotorTemp : Outport  Port=2
  MCU_PowerFdk : Outport  Port=3
  MCU1_idc : Outport  Port=4
  MCU_Udc : Outport  Port=5
  wires:
  MCU1/2(MCU1_MotorTemp_Out) -> MCU1_MotorTemp/1
  In1/1 -> MCU1/Enable
  MCU1/1(MCU1_ControlTemp_Out) -> MCU1_ControlTemp/1
  MCU1/4(MCU1_Idc_Out) -> MCU1_idc/1
  MCU1/5(MCU1_Udc_Out) -> MCU_Udc/1
  In2/1 -> MCU1/1(input)
  MCU1/3(MCU1_PowerFdk_Out) -> MCU_PowerFdk/1

== system six_plus_six_AcmsteeringV09_main/Data_input/MCU1_4 ==
  In1 : Inport
  In2 : Inport  Port=2
  Trigger : TriggerPort  TriggerType=function-call  PortDimensions=1
  MCU1 : Subsystem
  MCU1_ControlTemp : Outport
  MCU1_MotorTemp : Outport  Port=2
  MCU_PowerFdk : Outport  Port=3
  MCU1_idc : Outport  Port=4
  MCU_Udc : Outport  Port=5
  wires:
  MCU1/2(MCU1_MotorTemp_Out) -> MCU1_MotorTemp/1
  In1/1 -> MCU1/Enable
  MCU1/1(MCU1_ControlTemp_Out) -> MCU1_ControlTemp/1
  MCU1/4(MCU1_Idc_Out) -> MCU1_idc/1
  MCU1/5(MCU1_Udc_Out) -> MCU_Udc/1
  In2/1 -> MCU1/1(input)
  MCU1/3(MCU1_PowerFdk_Out) -> MCU_PowerFdk/1

== system six_plus_six_AcmsteeringV09_main/Data_input/MCU1_5 ==
  In1 : Inport
  In2 : Inport  Port=2
  Trigger : TriggerPort  TriggerType=function-call  PortDimensions=1
  MCU1 : Subsystem
  MCU1_ControlTemp : Outport
  MCU1_MotorTemp : Outport  Port=2
  MCU_PowerFdk : Outport  Port=3
  MCU1_idc : Outport  Port=4
  MCU_Udc : Outport  Port=5
  wires:
  MCU1/2(MCU1_MotorTemp_Out) -> MCU1_MotorTemp/1
  In1/1 -> MCU1/Enable
  MCU1/1(MCU1_ControlTemp_Out) -> MCU1_ControlTemp/1
  MCU1/4(MCU1_Idc_Out) -> MCU1_idc/1
  MCU1/5(MCU1_Udc_Out) -> MCU_Udc/1
  In2/1 -> MCU1/1(input)
  MCU1/3(MCU1_PowerFdk_Out) -> MCU_PowerFdk/1
